simulink model "BTcommLibrary"  (R2013b)
settings: Solver=ode45  StartTime=0.0  StopTime=10.0  RelTol=1e-3
libraries: embdlinuxlib x6, simulink x3
settings Model: Creator=mouyang  LastModifiedBy=mouyang

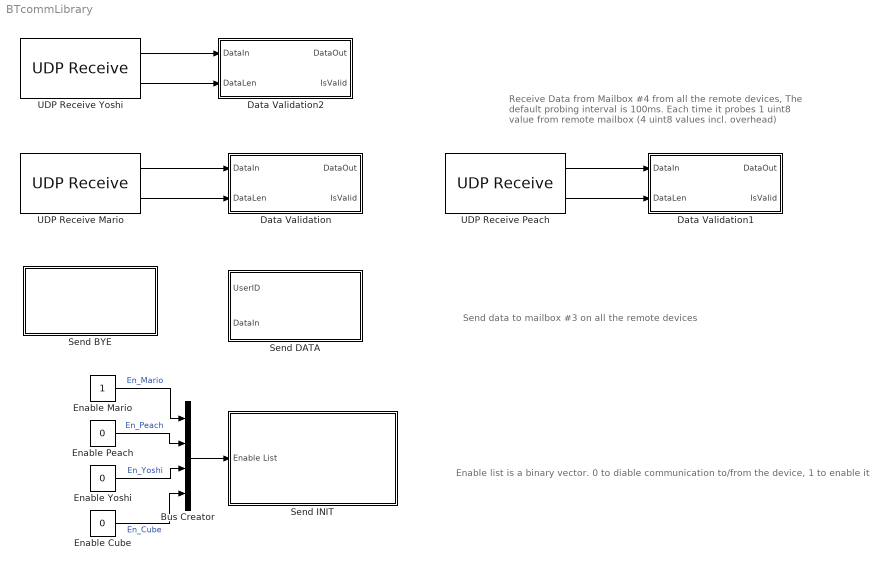
== system BTcommLibrary ==
  note: Enable list is a binary vector. 0 to diable communication to/from the device, 1 to enable it
  note: Send data to mailbox #3 on all the remote devices
  note: Receive Data from Mailbox #4 from all the remote devices,
      | The default probing interval is 100ms. Each time it probes 1
      | uint8 value from remote mailbox (4 uint8 values incl. overhead)
  Bus Creator : BusCreator
  Data Validation : Subsystem
  Data Validation1 : Subsystem
  Data Validation2 : Subsystem
  Enable Cube : Constant  Value=0  VectorParams1D=off  OutDataTypeStr=uint8
  Enable Mario : Constant  VectorParams1D=off  OutDataTypeStr=uint8
  Enable Peach : Constant  Value=0  VectorParams1D=off  OutDataTypeStr=uint8
  Enable Yoshi : Constant  Value=0  VectorParams1D=off  OutDataTypeStr=uint8
  Send BYE : Subsystem
      mask Display: disp('Send BYE')
  Send DATA : Subsystem
      mask Display: disp('Send DATA')
  Send INIT : Subsystem
      mask Display: disp('Send INIT')
  "UDP Receive Mario " : embdlinuxlib/UDP Receive  localURL='0.0.0.0'  localPort=35713  remoteURL='0.0.0.0'  remotePort=-1  recvBufferSize=8192  signalDatatype=uint8  dims=4  isVarSize=off  showBlockingTime=off  blockingTime=0  sampletime=0.1  blockPlatform=Raspberry Pi
  UDP Receive Peach : embdlinuxlib/UDP Receive  localURL='0.0.0.0'  localPort=35714  remoteURL='0.0.0.0'  remotePort=-1  recvBufferSize=8192  signalDatatype=uint8  dims=4  isVarSize=off  showBlockingTime=off  blockingTime=0  sampletime=0.1  blockPlatform=Raspberry Pi
  UDP Receive Yoshi : embdlinuxlib/UDP Receive  localURL='0.0.0.0'  localPort=35715  remoteURL='0.0.0.0'  remotePort=-1  recvBufferSize=8192  signalDatatype=uint8  dims=4  isVarSize=off  showBlockingTime=off  blockingTime=0  sampletime=0.1  blockPlatform=Raspberry Pi
  wires:
  UDP Receive Yoshi/1 -> Data Validation2/1(DataIn)
  UDP Receive Yoshi/2 -> Data Validation2/2(DataLen)
  "UDP Receive Mario "/2 -> Data Validation/2(DataLen)
  "UDP Receive Mario "/1 -> Data Validation/1(DataIn)
  UDP Receive Peach/2 -> Data Validation1/2(DataLen)
  UDP Receive Peach/1 -> Data Validation1/1(DataIn)
  Enable Mario/1 -> Bus Creator/1  "En_Mario"
  Enable Peach/1 -> Bus Creator/2  "En_Peach"
  Enable Yoshi/1 -> Bus Creator/3  "En_Yoshi"
  Enable Cube/1 -> Bus Creator/4  "En_Cube"
  Bus Creator/1 -> Send INIT/1(Enable List)

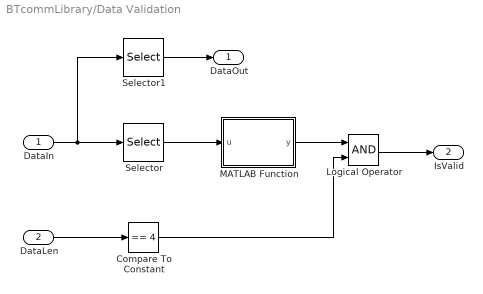
== system BTcommLibrary/Data Validation ==
  DataIn : Inport
  DataLen : Inport  Port=2
  Compare To Constant : simulink/Logic and Bit Operations/Compare To Constant  relop===  const=4  OutDataTypeStr=boolean
  Logical Operator : Logic  AllPortsSameDT=off  OutDataTypeStr=boolean
  MATLAB Function : MATLAB Function  TreatAsAtomicUnit=on
  Selector : Selector  InputPortWidth=4  IndexOptions=Index vector (dialog)  Indices=[1 2 3]  OutputSizes=1
  Selector1 : Selector  InputPortWidth=4  IndexOptions=Index vector (dialog)  Indices=[4]  OutputSizes=1
  DataOut : Outport
  IsValid : Outport  Port=2
  wires:
  Logical Operator/1 -> IsValid/1
  Compare To Constant/1 -> Logical Operator/2
  MATLAB Function/1(y) -> Logical Operator/1
  DataIn/1 -> Selector1/1, Selector/1
  Selector1/1 -> DataOut/1
  DataLen/1 -> Compare To Constant/1
  Selector/1 -> MATLAB Function/1(u)

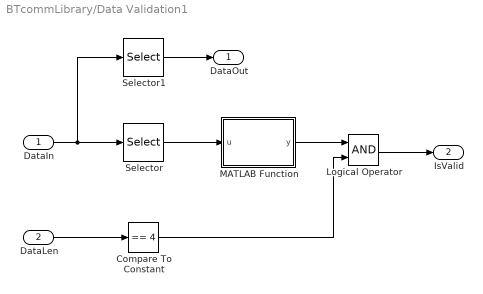
== system BTcommLibrary/Data Validation1 ==
  DataIn : Inport
  DataLen : Inport  Port=2
  Compare To Constant : simulink/Logic and Bit Operations/Compare To Constant  relop===  const=4  OutDataTypeStr=boolean
  Logical Operator : Logic  AllPortsSameDT=off  OutDataTypeStr=boolean
  MATLAB Function : MATLAB Function  TreatAsAtomicUnit=on
  Selector : Selector  InputPortWidth=4  IndexOptions=Index vector (dialog)  Indices=[1 2 3]  OutputSizes=1
  Selector1 : Selector  InputPortWidth=4  IndexOptions=Index vector (dialog)  Indices=[4]  OutputSizes=1
  DataOut : Outport
  IsValid : Outport  Port=2
  wires:
  Selector/1 -> MATLAB Function/1(u)
  DataLen/1 -> Compare To Constant/1
  Selector1/1 -> DataOut/1
  DataIn/1 -> Selector/1, Selector1/1
  MATLAB Function/1(y) -> Logical Operator/1
  Compare To Constant/1 -> Logical Operator/2
  Logical Operator/1 -> IsValid/1

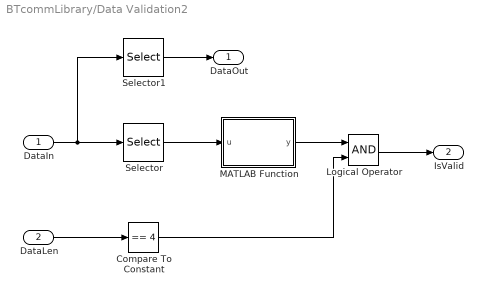
== system BTcommLibrary/Data Validation2 ==
  DataIn : Inport
  DataLen : Inport  Port=2
  Compare To Constant : simulink/Logic and Bit Operations/Compare To Constant  relop===  const=4  OutDataTypeStr=boolean
  Logical Operator : Logic  AllPortsSameDT=off  OutDataTypeStr=boolean
  MATLAB Function : MATLAB Function  TreatAsAtomicUnit=on
  Selector : Selector  InputPortWidth=4  IndexOptions=Index vector (dialog)  Indices=[1 2 3]  OutputSizes=1
  Selector1 : Selector  InputPortWidth=4  IndexOptions=Index vector (dialog)  Indices=[4]  OutputSizes=1
  DataOut : Outport
  IsValid : Outport  Port=2
  wires:
  Logical Operator/1 -> IsValid/1
  Compare To Constant/1 -> Logical Operator/2
  MATLAB Function/1(y) -> Logical Operator/1
  DataIn/1 -> Selector1/1, Selector/1
  Selector1/1 -> DataOut/1
  DataLen/1 -> Compare To Constant/1
  Selector/1 -> MATLAB Function/1(u)

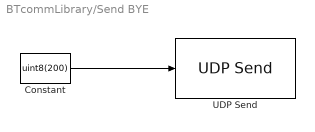
== system BTcommLibrary/Send BYE ==
  Constant : Constant  Value=uint8(200)  VectorParams1D=off
      settings: SamplingMode=Frame based
  UDP Send : embdlinuxlib/UDP Send  remoteURL='127.0.0.1'  remotePort=35712  localURL='255.255.255.255'  localPortSource=Automatically determine  localPort=-1  sampletime=-1  blockPlatform=Raspberry Pi  separateLengthPort=0
  wires:
  Constant/1 -> UDP Send/1

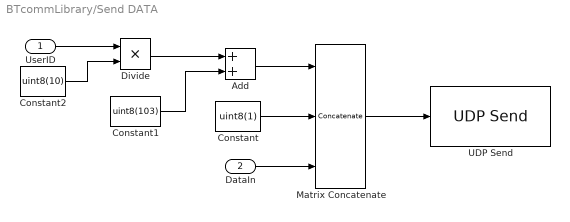
== system BTcommLibrary/Send DATA ==
  UserID : Inport
  DataIn : Inport  Port=2
  Add : Sum
  Constant : Constant  Value=uint8(1)  VectorParams1D=off
  Constant1 : Constant  Value=uint8(103)  VectorParams1D=off
  Constant2 : Constant  Value=uint8(10)  VectorParams1D=off
  Divide : Product  Inputs=**  OutDataTypeStr=uint8
  Matrix Concatenate : Concatenate  NumInputs=3  Mode=Multidimensional array
  UDP Send : embdlinuxlib/UDP Send  remoteURL='127.0.0.1'  remotePort=35712  localURL='255.255.255.255'  localPortSource=Automatically determine  localPort=-1  sampletime=-1  blockPlatform=Raspberry Pi  separateLengthPort=0
  wires:
  Matrix Concatenate/1 -> UDP Send/1
  DataIn/1 -> Matrix Concatenate/3
  Constant/1 -> Matrix Concatenate/2
  UserID/1 -> Divide/1
  Constant2/1 -> Divide/2
  Divide/1 -> Add/1
  Constant1/1 -> Add/2
  Add/1 -> Matrix Concatenate/1

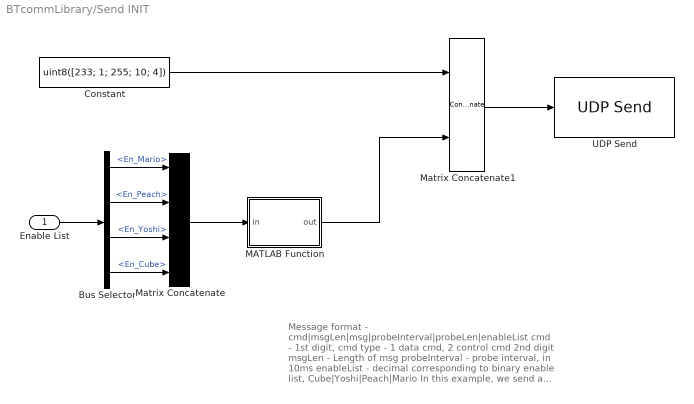
== system BTcommLibrary/Send INIT ==
  note: Message format -
      | cmd|msgLen|msg|probeInterval|probeLen|enableList
      | cmd - 1st digit, cmd type - 1 data cmd, 2 control cmd
      | 2nd digit
      | msgLen - Length of msg
      | probeInterval - probe interval, in 10ms
      | enableList - decimal corresponding to binary enable list,
      | Cube|Yoshi|Peach|Mario
      | In this example, we send a unint8 255
  Enable List : Inport
  Bus Selector : BusSelector  OutputSignals=En_Mario,En_Peach,En_Yoshi,En_Cube
  Constant : Constant  Value=uint8([233; 1; 255; 10; 4])  VectorParams1D=off
      settings: SamplingMode=Frame based
  MATLAB Function : MATLAB Function  TreatAsAtomicUnit=on
  Matrix Concatenate : Concatenate  NumInputs=4  ConcatenateDimension=2
  Matrix Concatenate1 : Concatenate  Mode=Multidimensional array
  UDP Send : embdlinuxlib/UDP Send  remoteURL='127.0.0.1'  remotePort=35712  localURL='255.255.255.255'  localPortSource=Automatically determine  localPort=-1  sampletime=-1  blockPlatform=Raspberry Pi  separateLengthPort=0
  wires:
  Matrix Concatenate/1 -> MATLAB Function/1(in)
  Matrix Concatenate1/1 -> UDP Send/1
  Constant/1 -> Matrix Concatenate1/1
  MATLAB Function/1(out) -> Matrix Concatenate1/2
  Enable List/1 -> Bus Selector/1
  Bus Selector/3 -> Matrix Concatenate/3  "<En_Yoshi>"
  Bus Selector/4 -> Matrix Concatenate/4  "<En_Cube>"
  Bus Selector/2 -> Matrix Concatenate/2  "<En_Peach>"
  Bus Selector/1 -> Matrix Concatenate/1  "<En_Mario>"

== matlab function BTcommLibrary/Data Validation2/MATLAB Function ==
  data: u input; y output
function y = fcn(u)
%#codegen

y = isequal(u,[2; 0; 4]);

== matlab function BTcommLibrary/Send INIT/MATLAB Function ==
  data: in input; out output uint8
function out = fcn(in)
%#codegen

out = uint8(bi2de(in.'));

== matlab function BTcommLibrary/Data Validation1/MATLAB Function ==
  data: u input; y output
function y = fcn(u)
%#codegen

y = isequal(u,[2; 0; 4]);

== matlab function BTcommLibrary/Data Validation/MATLAB Function ==
  data: u input; y output
function y = fcn(u)
%#codegen

y = isequal(u,[2; 0; 4]);
